simulink model "sampleModel1812"  (R2023a)
settings: Solver=VariableStepAuto  StartTime=0.0  StopTime=10.0  RelTol=1e-3
libraries: simulink x9, hdlsllib x2
settings Model: Creator=user1  LastModifiedBy=user1

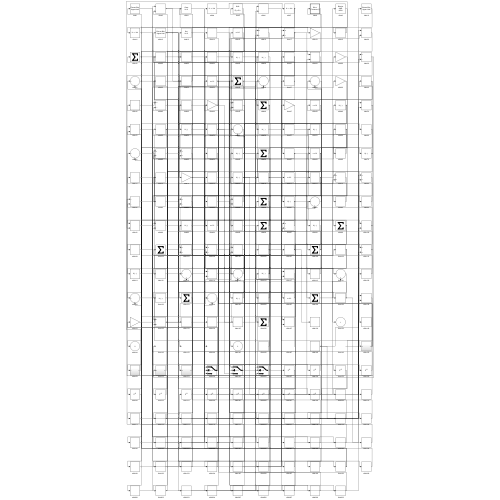
[thumbnail: Simulink's stored preview of the top-level diagram]
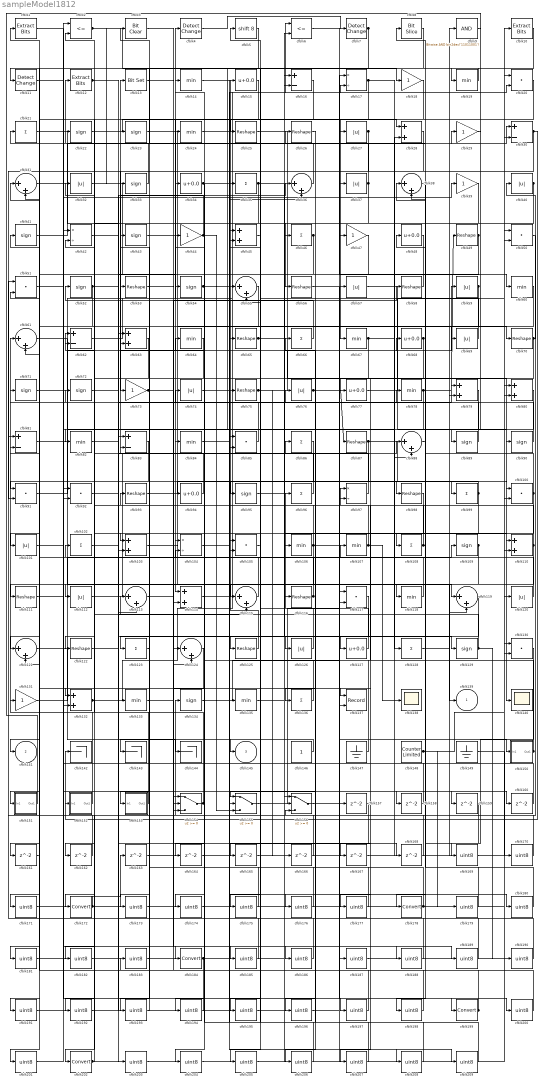
== system sampleModel1812 ==
  cfblk1 : simulink/Logic and Bit Operations/Extract Bits  bitsToExtract=Upper half  numBits=8  bitIdxRange=[0 7]  outScalingMode=Preserve fixed-point scaling
      settings: LibrarySourceBlock=|
      | hdlsllib/Logic and Bit
      | Operations/Extract Bits
  cfblk10 : simulink/Logic and Bit Operations/Extract Bits  bitsToExtract=Upper half  numBits=8  bitIdxRange=[0 7]  outScalingMode=Preserve fixed-point scaling
      settings: LibrarySourceBlock=|
      | hdlsllib/Logic and Bit
      | Operations/Extract Bits
  cfblk{20,50..51,85,91..92,100,105,117,130} (10 alike) : DotProduct  OutDataTypeStr=Inherit: Inherit via internal rule
  cfblk{27,32,37,40,57,59,69,74,76,101,112,120,126} (13 alike) : Abs  SaturateOnIntegerOverflow=off
  cfblk{21,35,46,66,86,96,99,102,108,123,128,136} (12 alike) : Sum  Inputs=+
  cfblk{28,45,63,79..80,103,110,114,132} (9 alike) : Sum
  cfblk{17,42,97,104} (4 alike) : Product  Inputs=*/  RndMeth=Zero  SaturateOnIntegerOverflow=on
  cfblk{14,19,24,60,64,67,78,82,84,106..107,118,133,135} (14 alike) : MinMax
  cfblk{22..23,33,41,43,52,54,71..72,89..90,95,109,129,134} (15 alike) : Signum
  cfblk11 : simulink/Logic and Bit Operations/Detect Change  vinit=0  OutDataTypeStr=boolean
      settings: LibrarySourceBlock=|
      | hdlsllib/Logic and Bit
      | Operations/Detect
      | Change
  cfblk{25..26,49,53,56,58,65,70,75,87,93,98,111,116,122,125} (16 alike) : Reshape
  cfblk{31,36,38,55,61,88,113,115,119,121,124} (11 alike) : Sum  Inputs=|++
  cfblk12 : simulink/Logic and Bit Operations/Extract Bits  bitsToExtract=Upper half  numBits=8  bitIdxRange=[0 7]  outScalingMode=Preserve fixed-point scaling
      settings: LibrarySourceBlock=|
      | hdlsllib/Logic and Bit
      | Operations/Extract Bits
  cfblk{15,34,48,68,77,94,127} (7 alike) : Bias  Bias=0.0  SaturateOnIntegerOverflow=off
  cfblk13 : simulink/Logic and Bit Operations/Bit Set  iBit=0
      settings: LibrarySourceBlock=|
      | hdlsllib/Logic and Bit
      | Operations/Bit Set
  cfblk{18,29,39,44,47,73,131} (7 alike) : Gain
  cfblk137 : Record  FileSettingsInternal="{\"entries\":[{\"content\":{\"excelSettings\":{\"content\":{},\"type\":\"Streamout.ExcelSettings\"}},\"type\":\"Streamout.FileSettingStorage\",\"uuid\":\"\"}],\"packageUris\":[\"http:\\/\\/schema.mathworks.com\\/mf0\\/streamout_blocks\\/R2020a\"],\"version\":\"1.0\"}"  Layout=[1 1]  SignalsInternal="{\"entries\":[{\"content\":{\"signals\":[{\"content\":{\"blockPath\":[],\"dimensions\":[1],\"domain\":\"\",\"lineColor\":\"#a2142f\",\"plots\":[1],\"port\":1,\"sid\":[\"\"],\"signalID\":4255,\"signalName\":\"cfblk98\"},\"type\":\"RecordBlkView.Signal\",\"uuid\":\"\"},{\"content\":{\"blockPath\":[],\"dimensions\":[1],\"domain\":\"\",\"lineColor\":\"#139fff\",\"plots\":[1],\"port\":2,\"sid\":[\"\"],\"signalID\":4259,\"signalName\":\"cfblk13\"},\"type\":\"RecordBlkView.Signal\",\"uuid\":\"\"}]},\"type\":\"RecordBlkView.InputSignals\",\"uuid\":\"\"}],\"packageUris\":[\"http:\\/\\/schema.mathworks.com\\/mf0\\/streamout_blocks\\/R2020a\"],\"version\":\"1.0\"}"  VisualizationBindings="{\"xyplotplugin\":{\"info\":[{\"series\":[{\"bindingParametersList\":[{\"parameter\":\"X-Axis\",\"signalID\":4255,\"signalName\":\"cfblk98\"},{\"parameter\":\"Y-Axis\",\"signalID\":4259,\"signalName\":\"cfblk13\"}],\"seriesID\":22271}],\"subplotID\":1}]}}"  CompatibilityTag=XY  st=-1
  cfblk138 : Scope
  cfblk140 : Scope
  cfblk142 : Terminator
  cfblk143 : Terminator
  cfblk144 : Terminator
  cfblk146 : Constant  SampleTime=-1
  cfblk147 : Ground
  cfblk148 : hdlsllib/Sources/Counter Limited  uplimit=7  tsamp=-1
  cfblk149 : Ground
  cfblk150 : Subsystem
      settings: LibrarySourceBlock=|
      | hdlsllib/Ports &
      | Subsystems/Subsystem
  cfblk151 : Subsystem
      settings: LibrarySourceBlock=|
      | hdlsllib/Ports &
      | Subsystems/Subsystem
  cfblk152 : Subsystem
      settings: LibrarySourceBlock=|
      | hdlsllib/Ports &
      | Subsystems/Subsystem
  cfblk153 : Subsystem
      settings: LibrarySourceBlock=|
      | hdlsllib/Ports &
      | Subsystems/Subsystem
  cfblk154 : Switch  SaturateOnIntegerOverflow=off  InputSameDT=off
  cfblk155 : Switch  SaturateOnIntegerOverflow=off  InputSameDT=off
  cfblk156 : Switch  SaturateOnIntegerOverflow=off  InputSameDT=off
  cfblk{157..168} (12 alike) : Delay  SampleTime=1
  cfblk{16,30,62,81,83} (5 alike) : Sum  Inputs=+-
  cfblk{169..171,173..177,179..183,185..198,200..201,203..209} (36 alike) : DataTypeConversion  OutDataTypeStr=uint8  SaturateOnIntegerOverflow=off  RndMeth=Floor
  cfblk{172,178,184,199,202} (5 alike) : DataTypeConversion  SaturateOnIntegerOverflow=off  RndMeth=Floor
  cfblk2 : RelationalOperator  Operator=<=  OutDataTypeStr=boolean  InputSameDT=off
  cfblk3 : simulink/Logic and Bit Operations/Bit Clear  iBit=0
      settings: LibrarySourceBlock=|
      | hdlsllib/Logic and Bit
      | Operations/Bit Clear
  cfblk4 : simulink/Logic and Bit Operations/Detect Change  vinit=0  OutDataTypeStr=boolean
      settings: LibrarySourceBlock=|
      | hdlsllib/Logic and Bit
      | Operations/Detect
      | Change
  cfblk5 : ArithShift  BitShiftNumber=8
  cfblk6 : RelationalOperator  Operator=<=  OutDataTypeStr=boolean  InputSameDT=off
  cfblk7 : simulink/Logic and Bit Operations/Detect Change  vinit=0  OutDataTypeStr=boolean
      settings: LibrarySourceBlock=|
      | hdlsllib/Logic and Bit
      | Operations/Detect
      | Change
  cfblk8 : hdlsllib/Logic and Bit Operations/Bit Slice  lidx=7  ridx=0
  cfblk9 : simulink/Logic and Bit Operations/Bitwise Operator  logicop=AND  UseBitMask=on  BitMask=bin2dec('11011001')  BitMaskRealWorld=Stored Integer
      settings: LibrarySourceBlock=|
      | hdlsllib/Logic and Bit
      | Operations/Bitwise
      | Operator
  cfblk139 : Outport  VectorParamsAs1DForOutWhenUnconnected=off
  cfblk141 : Outport  Port=2  VectorParamsAs1DForOutWhenUnconnected=off
  cfblk145 : Outport  Port=3  VectorParamsAs1DForOutWhenUnconnected=off
  wires:
  cfblk89/1 -> cfblk15/1
  cfblk112/1 -> cfblk86/1
  cfblk7/1 -> cfblk155/1, cfblk141/1
  cfblk25/1 -> cfblk140/1
  cfblk50/1 -> cfblk134/1
  cfblk22/1 -> cfblk28/1
  cfblk96/1 -> cfblk13/1
  cfblk57/1 -> cfblk90/1
  cfblk46/1 -> cfblk73/1, cfblk165/1
  cfblk72/1 -> cfblk36/1
  cfblk40/1 -> cfblk56/1, cfblk145/1
  cfblk20/1 -> cfblk114/1
  cfblk67/1 -> cfblk110/1, cfblk162/1
  cfblk23/1 -> cfblk155/2
  cfblk28/1 -> cfblk123/1
  cfblk43/1 -> cfblk70/1
  cfblk114/1 -> cfblk6/1
  cfblk131/1 -> cfblk107/1
  cfblk133/1 -> cfblk58/1
  cfblk126/1 -> cfblk96/1
  cfblk71/1 -> cfblk119/1
  cfblk154/1 -> cfblk61/1, cfblk81/2
  cfblk113/1 -> cfblk109/1
  cfblk125/1 -> cfblk65/1
  cfblk77/1 -> cfblk10/1
  cfblk34/1 -> cfblk36/2, cfblk174/1, cfblk176/1
  cfblk100/1 -> cfblk21/1, cfblk132/1
  cfblk66/1 -> cfblk52/1
  cfblk135/1 -> cfblk6/2
  cfblk52/1 -> cfblk101/1, cfblk34/1
  cfblk127/1 -> cfblk102/1
  cfblk30/1 -> cfblk142/1, cfblk206/1
  cfblk27/1 -> cfblk53/1, cfblk91/2
  cfblk115/1 -> cfblk61/2
  cfblk17/1 -> cfblk111/1, cfblk88/2, cfblk112/1
  cfblk18/1 -> cfblk67/1
  cfblk147/1 -> cfblk74/1
  cfblk91/1 -> cfblk30/1
  cfblk85/1 -> cfblk71/1
  cfblk136/1 -> cfblk85/1
  cfblk132/1 -> cfblk9/1, cfblk115/2
  cfblk81/1 -> cfblk68/1
  cfblk8/1 -> cfblk25/1
  cfblk44/1 -> cfblk23/1, cfblk155/3
  cfblk82/1 -> cfblk78/1
  cfblk78/1 -> cfblk49/1, cfblk154/2, cfblk132/2
  cfblk92/1 -> cfblk199/1
  cfblk65/1 -> cfblk129/1, cfblk17/2
  cfblk107/1 -> cfblk55/1, cfblk138/1
  cfblk69/1 -> cfblk5/1
  cfblk110/1 -> cfblk64/1, cfblk154/3
  cfblk54/1 -> cfblk35/1, cfblk135/1
  cfblk32/1 -> cfblk114/2
  cfblk99/1 -> cfblk91/1, cfblk177/1, cfblk204/1
  cfblk12/1 -> cfblk54/1, cfblk127/1, cfblk168/1
  cfblk16/1 -> cfblk202/1
  cfblk62/1 -> cfblk4/1
  cfblk70/1 -> cfblk125/1, cfblk40/1
  cfblk33/1 -> cfblk12/1
  cfblk93/1 -> cfblk98/1
  cfblk98/1 -> cfblk137/1
  cfblk103/1 -> cfblk139/1
  cfblk3/1 -> cfblk94/1
  cfblk120/1 -> cfblk62/1
  cfblk75/1 -> cfblk59/1, cfblk37/1, cfblk166/1
  cfblk48/1 -> cfblk104/1
  cfblk4/1 -> cfblk7/1
  cfblk39/1 -> cfblk84/1
  cfblk2/1 -> cfblk18/1, cfblk33/1
  cfblk87/1 -> cfblk99/1, cfblk161/1
  cfblk15/1 -> cfblk121/1
  cfblk76/1 -> cfblk87/1, cfblk150/1(In1)
  cfblk97/1 -> cfblk75/1
  cfblk58/1 -> cfblk57/1
  cfblk5/1 -> cfblk103/1
  cfblk106/1 -> cfblk79/1, cfblk62/2, cfblk164/1
  cfblk35/1 -> cfblk82/1, cfblk100/1
  cfblk36/1 -> cfblk3/1
  cfblk68/1 -> cfblk77/1, cfblk167/1
  cfblk121/1 -> cfblk144/1
  cfblk146/1 -> cfblk143/1
  cfblk123/1 -> cfblk153/1(In1)
  cfblk41/1 -> cfblk29/1
  cfblk155/1 -> cfblk47/1
  cfblk128/1 -> cfblk119/2
  cfblk152/1(Out1) -> cfblk41/1
  cfblk151/1(Out1) -> cfblk19/1
  cfblk95/1 -> cfblk108/1
  cfblk51/1 -> cfblk184/1
  cfblk29/1 -> cfblk69/1
  cfblk148/1 -> cfblk120/1, cfblk179/1
  cfblk26/1 -> cfblk46/1
  cfblk88/1 -> cfblk48/1
  cfblk74/1 -> cfblk20/2
  cfblk116/1 -> cfblk44/1, cfblk32/1, cfblk43/1
  cfblk101/1 -> cfblk39/1
  cfblk24/1 -> cfblk126/1
  cfblk31/1 -> cfblk113/2
  cfblk86/1 -> cfblk103/2
  cfblk102/1 -> cfblk63/1
  cfblk6/1 -> cfblk60/1
  cfblk73/1 -> cfblk188/1, cfblk189/1
  cfblk38/1 -> cfblk178/1
  cfblk134/1 -> cfblk17/1
  cfblk21/1 -> cfblk133/1
  cfblk49/1 -> cfblk115/1, cfblk136/1
  cfblk9/1 -> cfblk89/1
  cfblk37/1 -> cfblk85/2, cfblk26/1
  cfblk10/1 -> cfblk95/1
  cfblk108/1 -> cfblk97/1, cfblk8/1
  cfblk109/1 -> cfblk151/1(In1), cfblk207/1
  cfblk59/1 -> cfblk121/2, cfblk118/1
  cfblk61/1 -> cfblk128/1
  cfblk94/1 -> cfblk2/2
  cfblk90/1 -> cfblk55/2
  cfblk129/1 -> cfblk42/2, cfblk190/1
  cfblk122/1 -> cfblk88/1
  cfblk13/1 -> cfblk137/2
  cfblk19/1 -> cfblk11/1
  cfblk118/1 -> cfblk24/1
  cfblk150/1(Out1) -> cfblk22/1, cfblk63/2, cfblk97/2
  cfblk153/1(Out1) -> cfblk72/1
  cfblk63/1 -> cfblk122/1
  cfblk80/1 -> cfblk172/1
  cfblk53/1 -> cfblk158/1
  cfblk158/1 -> cfblk42/1
  cfblk111/1 -> cfblk159/1
  cfblk104/1 -> cfblk160/1
  cfblk160/1 -> cfblk113/1
  cfblk162/1 -> cfblk2/1
  cfblk163/1 -> cfblk79/2
  cfblk165/1 -> cfblk110/2
  cfblk166/1 -> cfblk81/1
  cfblk167/1 -> cfblk28/2
  cfblk168/1 -> cfblk31/2
  cfblk130/1 -> cfblk169/1
  cfblk169/1 -> cfblk20/1
  cfblk149/1 -> cfblk170/1
  cfblk170/1 -> cfblk130/1
  cfblk47/1 -> cfblk171/1
  cfblk171/1 -> cfblk130/2
  cfblk172/1 -> cfblk163/1, cfblk100/2
  cfblk79/1 -> cfblk173/1
  cfblk173/1 -> cfblk80/1
  cfblk174/1 -> cfblk80/2
  cfblk105/1 -> cfblk175/1
  cfblk175/1 -> cfblk93/1
  cfblk176/1 -> cfblk105/1
  cfblk177/1 -> cfblk105/2
  cfblk178/1 -> cfblk76/1, cfblk30/2
  cfblk179/1 -> cfblk38/1
  cfblk84/1 -> cfblk180/1
  cfblk180/1 -> cfblk38/2
  cfblk124/1 -> cfblk181/1
  cfblk181/1 -> cfblk106/1
  cfblk64/1 -> cfblk182/1
  cfblk182/1 -> cfblk124/1
  cfblk183/1 -> cfblk124/2
  cfblk184/1 -> cfblk183/1, cfblk104/2, cfblk209/1
  cfblk11/1 -> cfblk185/1
  cfblk185/1 -> cfblk51/1
  cfblk164/1 -> cfblk186/1
  cfblk186/1 -> cfblk51/2
  cfblk156/1 -> cfblk187/1
  cfblk187/1 -> cfblk50/1
  cfblk188/1 -> cfblk156/1
  cfblk189/1 -> cfblk156/2
  cfblk190/1 -> cfblk156/3
  cfblk83/1 -> cfblk191/1
  cfblk191/1 -> cfblk157/1
  cfblk55/1 -> cfblk192/1
  cfblk192/1 -> cfblk83/1
  cfblk119/1 -> cfblk193/1
  cfblk193/1 -> cfblk83/2
  cfblk117/1 -> cfblk194/1
  cfblk194/1 -> cfblk131/1
  cfblk157/1 -> cfblk195/1
  cfblk195/1 -> cfblk117/1
  cfblk60/1 -> cfblk196/1
  cfblk196/1 -> cfblk117/2
  cfblk1/1 -> cfblk197/1
  cfblk197/1 -> cfblk31/1
  cfblk159/1 -> cfblk198/1
  cfblk198/1 -> cfblk1/1
  cfblk199/1 -> cfblk154/1, cfblk66/1
  cfblk56/1 -> cfblk200/1
  cfblk200/1 -> cfblk92/1
  cfblk161/1 -> cfblk201/1
  cfblk201/1 -> cfblk92/2
  cfblk202/1 -> cfblk152/1(In1), cfblk27/1
  cfblk42/1 -> cfblk203/1
  cfblk203/1 -> cfblk16/1
  cfblk204/1 -> cfblk16/2
  cfblk45/1 -> cfblk205/1
  cfblk205/1 -> cfblk50/2
  cfblk206/1 -> cfblk45/1
  cfblk207/1 -> cfblk45/2
  cfblk14/1 -> cfblk208/1
  cfblk208/1 -> cfblk116/1
  cfblk209/1 -> cfblk14/1

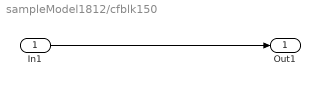
== system sampleModel1812/cfblk150 ==
  In1 : Inport
  Out1 : Outport
  wires:
  In1/1 -> Out1/1

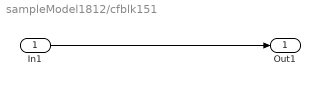
== system sampleModel1812/cfblk151 ==
  In1 : Inport
  Out1 : Outport
  wires:
  In1/1 -> Out1/1

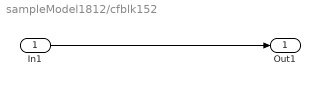
== system sampleModel1812/cfblk152 ==
  In1 : Inport
  Out1 : Outport
  wires:
  In1/1 -> Out1/1

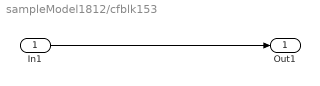
== system sampleModel1812/cfblk153 ==
  In1 : Inport
  Out1 : Outport
  wires:
  In1/1 -> Out1/1
